simulink model "model_thermal_gust"  (R2020b)
settings: configuration reference "Configuration" (kept outside this file)
settings Model: Creator=C:\Users\Dogukan  LastModifiedBy=dogukan
settings ConfigSetRef: SourceName=Configuration  SourceLocation=Base Workspace

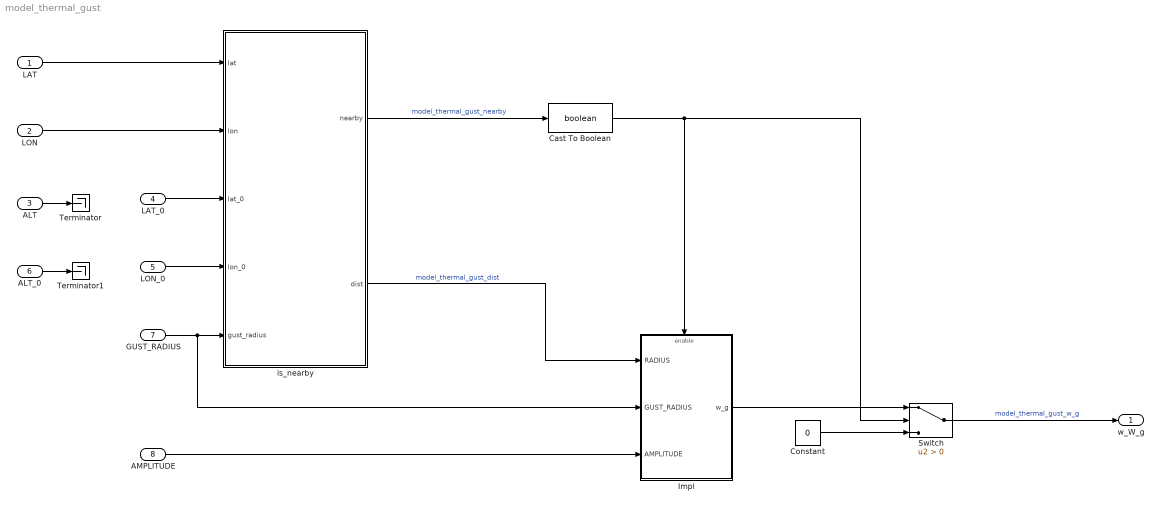
== system model_thermal_gust ==
  LAT : Inport  OutDataTypeStr=double
  LON : Inport  Port=2  OutDataTypeStr=double
  ALT : Inport  Port=3  OutDataTypeStr=double
  LAT_0 : Inport  Port=4  OutDataTypeStr=double
  LON_0 : Inport  Port=5  OutDataTypeStr=double
  ALT_0 : Inport  Port=6  OutDataTypeStr=double
  GUST_RADIUS : Inport  Port=7  OutDataTypeStr=double
  AMPLITUDE : Inport  Port=8  OutDataTypeStr=double
  Cast To Boolean : DataTypeConversion  OutDataTypeStr=boolean
  Constant : Constant  Value=0
  Impl : Subsystem  TreatAsAtomicUnit=on
  Switch : Switch  Criteria=u2 > Threshold
  Terminator : Terminator
  Terminator1 : Terminator
  is_nearby : MATLAB Function  TreatAsAtomicUnit=on
  w_W_g : Outport  SignalName=w_W_g  OutDataTypeStr=double
  wires:
  ALT/1 -> Terminator/1
  LAT/1 -> is_nearby/1(lat)
  LON/1 -> is_nearby/2(lon)
  LAT_0/1 -> is_nearby/3(lat_0)
  LON_0/1 -> is_nearby/4(lon_0)
  ALT_0/1 -> Terminator1/1
  GUST_RADIUS/1 -> Impl/2(GUST_RADIUS), is_nearby/5(gust_radius)
  is_nearby/1(nearby) -> Cast To Boolean/1  "model_thermal_gust_nearby"
  Cast To Boolean/1 -> Impl/Enable, Switch/2
  Switch/1 -> w_W_g/1  "model_thermal_gust_w_g"
  Constant/1 -> Switch/3
  Impl/1(w_g) -> Switch/1
  AMPLITUDE/1 -> Impl/3(AMPLITUDE)
  is_nearby/2(dist) -> Impl/1(RADIUS)  "model_thermal_gust_dist"

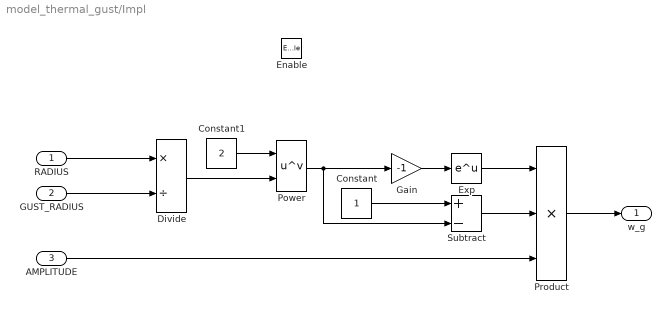
== system model_thermal_gust/Impl ==
  RADIUS : Inport  OutDataTypeStr=double
  GUST_RADIUS : Inport  Port=2  OutDataTypeStr=double
  AMPLITUDE : Inport  Port=3  OutDataTypeStr=double
  Enable : EnablePort
  Constant : Constant
  Constant1 : Constant  Value=2
  Divide : Product  Inputs=*/
  Exp : Math  SaturateOnIntegerOverflow=on
  Gain : Gain  Gain=-1
  Power : Math  Operator=pow  SaturateOnIntegerOverflow=on
  Product : Product  Inputs=3
  Subtract : Sum  Inputs=+-
  w_g : Outport  OutDataTypeStr=double
  wires:
  RADIUS/1 -> Divide/1
  GUST_RADIUS/1 -> Divide/2
  Product/1 -> w_g/1
  AMPLITUDE/1 -> Product/3
  Constant/1 -> Subtract/1
  Divide/1 -> Power/2
  Subtract/1 -> Product/2
  Constant1/1 -> Power/1
  Power/1 -> Gain/1, Subtract/2
  Gain/1 -> Exp/1
  Exp/1 -> Product/1

== matlab function model_thermal_gust/is_nearby ==
  data: lat input; nearby output; lon input; lat_0 input; lon_0 input; dist output; gust_radius input
% model_thermal_gust
function [nearby, dist] = is_nearby(lat, lon, lat_0, lon_0, gust_radius)
    % Units:
    % [lat] = rad
    % [lon] = rad
    % [lat_0] = rad
    % [lon_0] = rad
    % [height_0] = m
    % [gust_width] = m
    % Independet of altitude, phenomena is available on all heights, because otherwise height distribution is needed

    % Option 1: doesn't support code gen
    % [arclen, az] = distance(lat, lon, lat0, lon0);
    % nearby = arclen < width;

    % Option 2: ¯\_(ツ)_/¯
    earth_radius = 6371000; % m
    delta_phi = lat - lat_0;
    delta_lambda = lon - lon_0;
    a = sin(delta_phi / 2) ^ 2 + cos(lat) * cos(lat_0) * sin(delta_lambda / 2) ^ 2;
    c = 2 * atan2(sqrt(a), sqrt(1 - a));
    dist = earth_radius * c;
    nearby = abs(dist) < gust_radius*2.5;

    % Option 3:
    % lat_0 = rad2deg(lat_0); % ned2lla needs lla in degrees
    % lon_0 = rad2deg(lon_0); % ned2lla needs lla in degrees

    % north_lla = ned2lla([gust_width/2, 0, 0], [lat_0, lon_0, alt_0], "flat");
    % north = deg2rad(north_lla(1)); % rad
    % south_lla = ned2lla([-gust_width/2, 0, 0], [lat_0, lon_0, alt_0], "flat");
    % south = deg2rad(south_lla(1)); % rad
    % inside_lat = (south < lat) & (lat < north);

    % east_lla = ned2lla([0, gust_width/2, 0], [lat_0, lon_0, alt_0], "flat");
    % east = deg2rad(east_lla(2)); % rad
    % west_lla = ned2lla([0, -gust_width/2, 0], [lat_0, lon_0, alt_0], "flat");
    % west = deg2rad(west_lla(2)); % rad
    % inside_lon = (west < lon) & (lon < east);

    % nearby = inside_lat & inside_lon;
end
